simulink model "version_rara"  (R2021a)
settings: Solver=VariableStepAuto  StartTime=0.0  StopTime=300  RelTol=1e-3
settings Model: Creator=jmata  LastModifiedBy=cgrc1

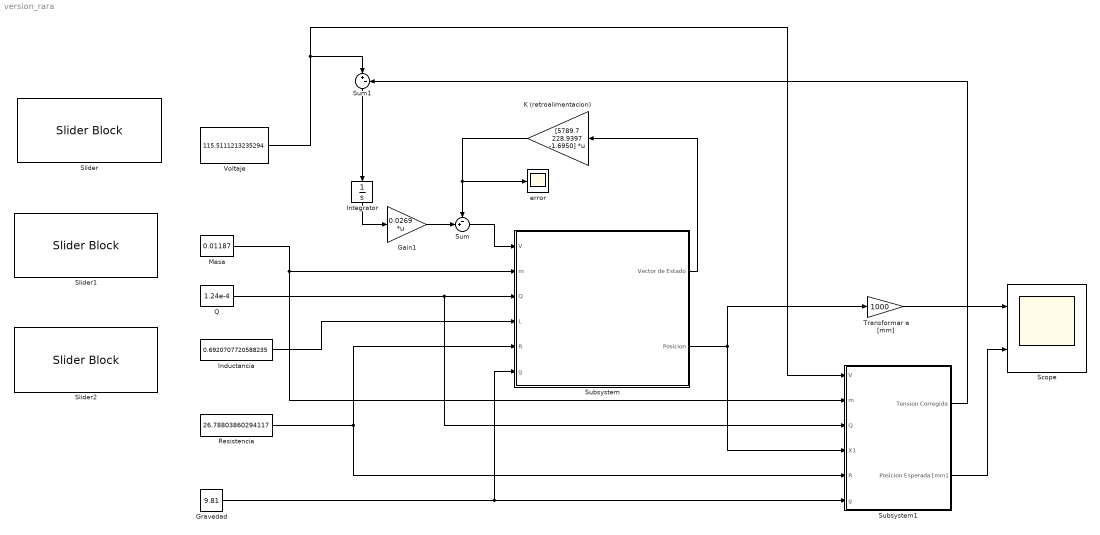
== system version_rara ==
  Gain1 : Gain  Gain=0.0269  Multiplication=Matrix(K*u)
  Gravedad : Constant  Value=9.81
  Inductancia : Constant  Value=0.6920707720588235
  Integrator : Integrator
  K (retroalimentacion) : Gain  Gain=[5789.7 228.9397 -1.6950]  Multiplication=Matrix(K*u)
  Masa : Constant  Value=0.01187
  Q : Constant  Value=1.24e-4
  Resistencia : Constant  Value=26.78803860294117
  Scope : Scope  NumInputPorts=2
  Slider : SliderBlock  ScaleMin=93.5  ScaleMax=126.5
  Slider1 : SliderBlock  ScaleMin=24.93  ScaleMax=30.47
  Slider2 : SliderBlock  ScaleMin=0.585  ScaleMax=0.715
  Subsystem : Subsystem
  Subsystem1 : Subsystem
  Sum : Sum  Inputs=-+|
  Sum1 : Sum  Inputs=|+-
  Transformar a [mm] : Gain  Gain=1000
  Voltaje : Constant  Value=115.5111213235294
  error : Scope
  wires:
  Masa/1 -> Subsystem/2(m), Subsystem1/2(m)
  Q/1 -> Subsystem/3(Q), Subsystem1/3(Q)
  Inductancia/1 -> Subsystem/4(L)
  Resistencia/1 -> Subsystem/5(R), Subsystem1/5(R)
  Gravedad/1 -> Subsystem/6(g), Subsystem1/6(g)
  Subsystem/1(Vector de Estado) -> K (retroalimentacion)/1
  K (retroalimentacion)/1 -> Sum/1, error/1
  Transformar a [mm]/1 -> Scope/1
  Subsystem/2(Posicion) -> Transformar a [mm]/1, Subsystem1/4(X1)
  Sum/1 -> Subsystem/1(V)
  Gain1/1 -> Sum/2
  Integrator/1 -> Gain1/1
  Sum1/1 -> Integrator/1
  Voltaje/1 -> Subsystem1/1(V), Sum1/1
  Subsystem1/1(Tension Corregida) -> Sum1/2
  Subsystem1/2("Posicion Esperada [mm] ") -> Scope/2

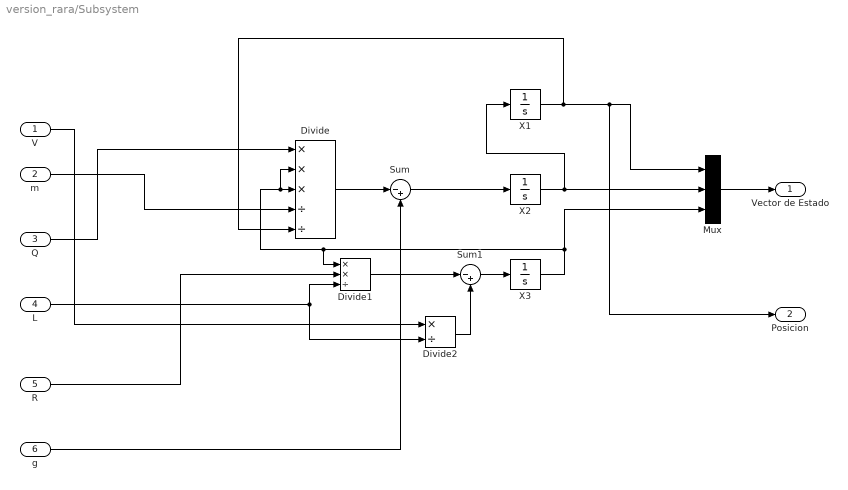
== system version_rara/Subsystem ==
  V : Inport
  m : Inport  Port=2
  Q : Inport  Port=3
  L : Inport  Port=4
  R : Inport  Port=5
  g : Inport  Port=6
  Divide : Product  Inputs=***//
  Divide1 : Product  Inputs=**/
  Divide2 : Product  Inputs=*/
  Mux : Mux  Inputs=3
  Sum : Sum  Inputs=|-+
  Sum1 : Sum  Inputs=|-+
  X1 : Integrator  InitialCondition=0.001
  X2 : Integrator
  X3 : Integrator
  Vector de Estado : Outport
  Posicion : Outport  Port=2
  wires:
  Divide/1 -> Sum/1
  Sum/1 -> X2/1
  L/1 -> Divide2/2, Divide1/3
  Sum1/1 -> X3/1
  X3/1 -> Mux/3, Divide1/1, Divide/2, Divide/3
  Divide2/1 -> Sum1/2
  X1/1 -> Posicion/1, Mux/1, Divide/5
  X2/1 -> Mux/2, X1/1
  g/1 -> Sum/2
  Divide1/1 -> Sum1/1
  m/1 -> Divide/4
  Q/1 -> Divide/1
  Mux/1 -> Vector de Estado/1
  R/1 -> Divide1/2
  V/1 -> Divide2/1

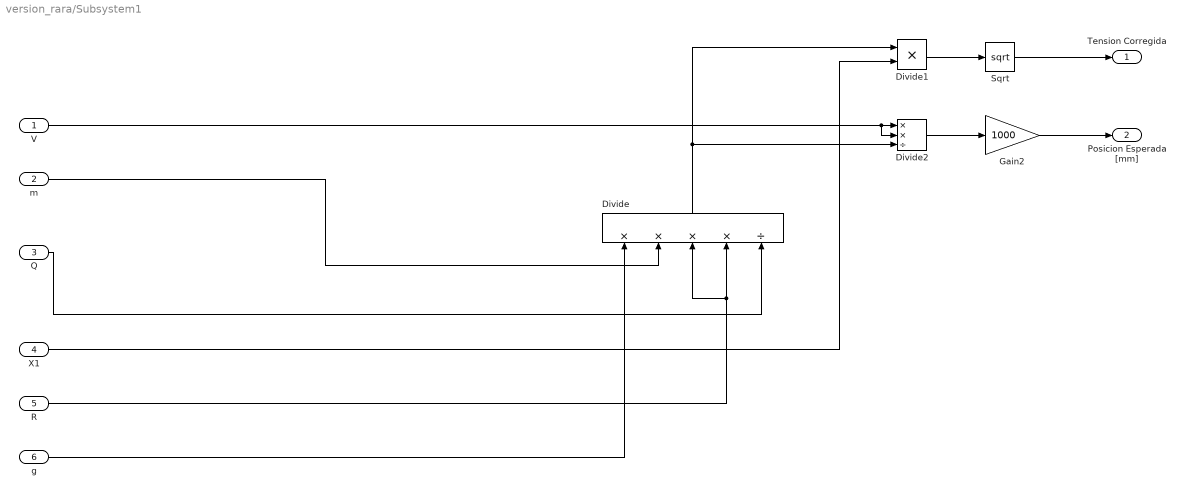
== system version_rara/Subsystem1 ==
  V : Inport
  m : Inport  Port=2
  Q : Inport  Port=3
  X1 : Inport  Port=4
  R : Inport  Port=5
  g : Inport  Port=6
  Divide : Product  Inputs=****/
  Divide1 : Product  Inputs=**
  Divide2 : Product  Inputs=**/
  Gain2 : Gain  Gain=1000
  Sqrt : Sqrt  SaturateOnIntegerOverflow=on
  Tension Corregida : Outport
  "Posicion Esperada [mm] " : Outport  Port=2
  wires:
  R/1 -> Divide/3, Divide/4
  X1/1 -> Divide1/2
  Divide1/1 -> Sqrt/1
  Divide2/1 -> Gain2/1
  Divide/1 -> Divide1/1, Divide2/3
  Q/1 -> Divide/5
  m/1 -> Divide/2
  Gain2/1 -> "Posicion Esperada [mm] "/1
  g/1 -> Divide/1
  Sqrt/1 -> Tension Corregida/1
  V/1 -> Divide2/2, Divide2/1
